simulink model "Hipotenso"  (R2023a)
settings: Solver=ode45  StartTime=0.0  StopTime=10  MaxStep=1E-3  RelTol=1e-3
libraries: slpidlib x1
settings Model: LastModifiedBy=diegt
settings DataIOCC: ReturnWorkspaceOutputs=off  TimeSaveName=t
settings DebuggingCC: AlgebraicLoopMsg=none  ArtificialAlgebraicLoopMsg=none  MaxConsecutiveZCsMsg=none  ModelReferenceExtraNoncontSigs=none  OperatingPointInterfaceChecksumMismatchMsg=none
settings RTWCC: GPUComputeCapability=5.0

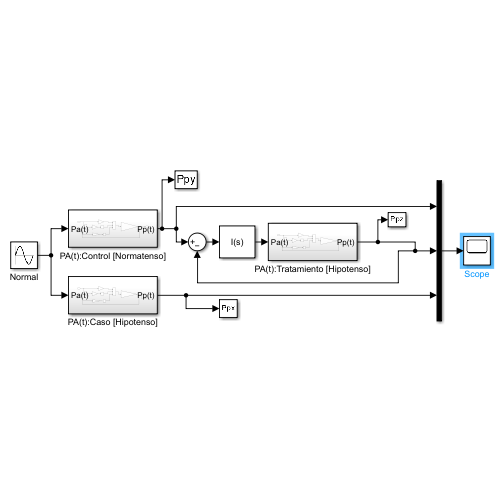
[thumbnail: Simulink's stored preview of the top-level diagram]
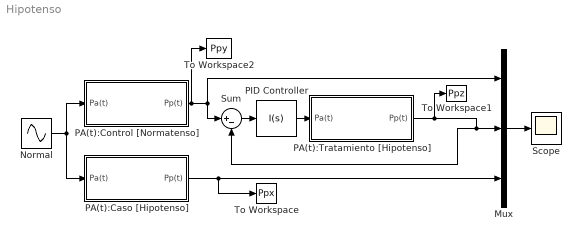
== system Hipotenso ==
  Mux : Mux  Inputs=3
  Normal : Sin  Bias=0.8  Frequency=((2*pi)*(95/60))
  PA(t):Caso [Hipotenso] : Subsystem
  PA(t):Control [Normatenso] : Subsystem
  PA(t):Tratamiento [Hipotenso] : Subsystem
  PID Controller : slpidlib/PID Controller  Controller=I  Form=Parallel  TimeDomain=Continuous-time  UseExternalTs=off  SampleTime=-1  IntegratorMethod=Forward Euler  FilterMethod=Forward Euler  ControllerParametersSource=internal  P=0  I=13686.5342163355  UseKiTs=off  D=0  N=100  UseFilter=on  TunerSelectOption=Transfer Function Based (PID Tuner App)  InitialConditionSource=internal  InitialConditionForIntegrator=0  InitialConditionForFilter=0  DifferentiatorICPrevScaledInput=0  ExternalReset=none  TrackingMode=off  Kt=1  LimitOutput=off  SatLimitsSource=internal  UpperSaturationLimit=inf  LowerSaturationLimit=-inf  LinearizeAsGain=on  AntiWindupMode=none  Kb=1  LimitIntegrator=off  UpperIntegratorSaturationLimit=inf  LowerIntegratorSaturationLimit=-inf  POutMin=[]  POutMax=[]  IOutMin=[]  IOutMax=[]  DOutMin=[]  DOutMax=[]  NOutMin=[]  NOutMax=[]  SumOutMin=[]  SumOutMax=[]  SaturationOutMin=[]  SaturationOutMax=[]  PParamMin=[]  PParamMax=[]  IParamMin=[]  IParamMax=[]  DParamMin=[]  DParamMax=[]  NParamMin=[]  NParamMax=[]  KbParamMin=[]  KbParamMax=[]  KtParamMin=[]  KtParamMax=[]  KbOutMin=[]  KbOutMax=[]  KtOutMin=[]  KtOutMax=[]  IntegratorOutMin=[]  IntegratorOutMax=[]  FilterOutMin=[]  FilterOutMax=[]  SumI1OutMin=[]  SumI1OutMax=[]  SumI2OutMin=[]  SumI2OutMax=[]  SumI3OutMin=[]  SumI3OutMax=[]  SumI4OutMin=[]  SumI4OutMax=[]  SumDOutMin=[]  SumDOutMax=[]  DifferentiatorOutMin=[]  DifferentiatorOutMax=[]  FilterDiffOutCoefMin=[]  FilterDiffOutCoefMax=[]  ReciprocalOutMin=[]  ReciprocalOutMax=[]  SumDenOutMin=[]  SumDenOutMax=[]  SumNumOutMin=[]  SumNumOutMax=[]  DivideOutMin=[]  DivideOutMax=[]  UdiffTsProdOutMin=[]  UdiffTsProdOutMax=[]  NTsProdOutMin=[]  NTsProdOutMax=[]  UintegralTsProdOutMin=[]  UintegralTsProdOutMax=[]  UngainTsProdOutMin=[]  UngainTsProdOutMax=[]  ClampingZeroOutDataTypeStr=Inherit: Inherit via back propagation  ClampingZeroOutMin=[]  ClampingZeroOutMax=[]  FilterDenConstantOutDataTypeStr=Inherit: Inherit via back propagation  FilterDenConstantOutMin=[]  FilterDenConstantOutMax=[]  PCopyOutDataTypeStr=Inherit: Inherit via back propagation  PCopyOutMin=[]  PCopyOutMax=[]  NCopyOutDataTypeStr=Inherit: Inherit via back propagation  NCopyOutMin=[]  NCopyOutMax=[]  IntegratorContinuousStateAttributes=''  IntegratorStateMustResolveToSignalObject=off  IntegratorRTWStateStorageClass=Auto  FilterContinuousStateAttributes=''  FilterStateMustResolveToSignalObject=off  FilterRTWStateStorageClass=Auto  ParallelPVariant=Disabled  IdealPVariant=Disabled  IVariant=InternalParameters  DVariant=Disabled  IntegratorVariant=Continuous  SatVariant=Disabled  AWVariant=Passthrough  PCopyVariant=Disabled  TRVariant=Disabled  FdbkBlocksVariant=Forward  IdealPFdbkVariant=Disabled  SatFdbkVariant=Disabled  DerivativeFilterVariant=Disabled  NVariant=Disabled  NCopyVariant=Disabled_SignalSpec  FilterICVariant=Disabled  IntegratorICVariant=InternalICs  ExternalResetVariant=Disabled  TRSumVariant=Passthrough  SumFdbkVariant=Disabled  SumVariant=Passthrough_I  TsampFilterVariant=InternalTs  TsampNgainVariant=Passthrough  TsampIntegralVariant=Disabled_SignalSpec  ExternalSaturationOutDataTypeStr=Inherit: Same as second input
  Scope : Scope
  Sum : Sum  Inputs=|+-
  To Workspace : ToWorkspace  VariableName=Ppx  SampleTime=-1
  To Workspace1 : ToWorkspace  VariableName=Ppz  SampleTime=-1
  To Workspace2 : ToWorkspace  VariableName=Ppy  SampleTime=-1
  wires:
  Mux/1 -> Scope/1
  Normal/1 -> PA(t):Caso [Hipotenso]/1(Pa(t)), PA(t):Control [Normatenso]/1(Pa(t))
  PA(t):Control [Normatenso]/1(Pp(t)) -> Sum/1, Mux/1, To Workspace2/1
  Sum/1 -> PID Controller/1
  PA(t):Caso [Hipotenso]/1(Pp(t)) -> Mux/3, To Workspace/1
  PID Controller/1 -> PA(t):Tratamiento [Hipotenso]/1(Pa(t))
  PA(t):Tratamiento [Hipotenso]/1(Pp(t)) -> To Workspace1/1, Mux/2, Sum/2

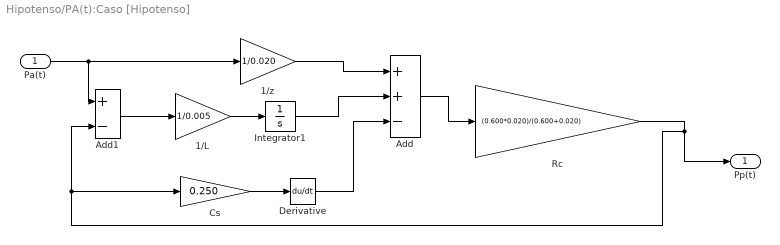
== system Hipotenso/PA(t):Caso [Hipotenso] ==
  Pa(t) : Inport
  1/L : Gain  Gain=1/0.005
  1/z : Gain  Gain=1/0.020
  Add : Sum  Inputs=++-
  Add1 : Sum  Inputs=+-
  Cs : Gain  Gain=0.250
  Derivative : Derivative
  Integrator1 : Integrator
  Rc : Gain  Gain=(0.600*0.020)/(0.600+0.020)
  Pp(t) : Outport
  wires:
  Pa(t)/1 -> Add1/1, 1/z/1
  1/z/1 -> Add/1
  Add1/1 -> 1/L/1
  Rc/1 -> Cs/1, Add1/2, Pp(t)/1
  Cs/1 -> Derivative/1
  Integrator1/1 -> Add/2
  1/L/1 -> Integrator1/1
  Derivative/1 -> Add/3
  Add/1 -> Rc/1

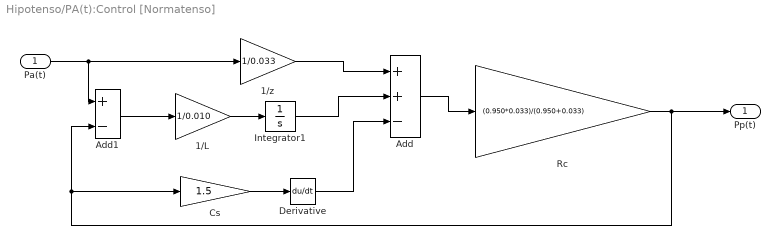
== system Hipotenso/PA(t):Control [Normatenso] ==
  Pa(t) : Inport
  1/L : Gain  Gain=1/0.010
  1/z : Gain  Gain=1/0.033
  Add : Sum  Inputs=++-
  Add1 : Sum  Inputs=+-
  Cs : Gain  Gain=1.5
  Derivative : Derivative
  Integrator1 : Integrator
  Rc : Gain  Gain=(0.950*0.033)/(0.950+0.033)
  Pp(t) : Outport
  wires:
  Pa(t)/1 -> Add1/1, 1/z/1
  1/z/1 -> Add/1
  Add/1 -> Rc/1
  Add1/1 -> 1/L/1
  Rc/1 -> Pp(t)/1, Cs/1, Add1/2
  Cs/1 -> Derivative/1
  Integrator1/1 -> Add/2
  1/L/1 -> Integrator1/1
  Derivative/1 -> Add/3

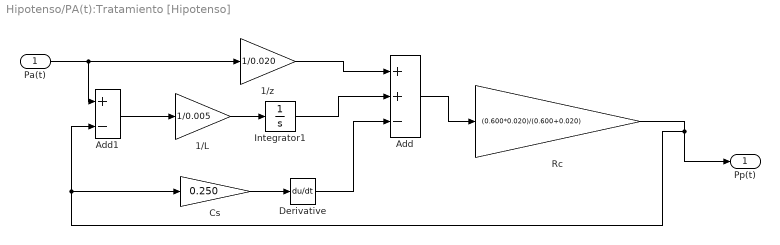
== system Hipotenso/PA(t):Tratamiento [Hipotenso] ==
  Pa(t) : Inport
  1/L : Gain  Gain=1/0.005
  1/z : Gain  Gain=1/0.020
  Add : Sum  Inputs=++-
  Add1 : Sum  Inputs=+-
  Cs : Gain  Gain=0.250
  Derivative : Derivative
  Integrator1 : Integrator
  Rc : Gain  Gain=(0.600*0.020)/(0.600+0.020)
  Pp(t) : Outport
  wires:
  Pa(t)/1 -> Add1/1, 1/z/1
  1/z/1 -> Add/1
  Add1/1 -> 1/L/1
  Rc/1 -> Cs/1, Add1/2, Pp(t)/1
  Cs/1 -> Derivative/1
  Integrator1/1 -> Add/2
  1/L/1 -> Integrator1/1
  Derivative/1 -> Add/3
  Add/1 -> Rc/1
